simulink model "Intersection_Sim_V23"  (R2024b)
settings: Solver=VariableStepAuto  StartTime=0.0  StopTime=5  RelTol=1e-3
settings Model: Creator=nelsenyoung  LastModifiedBy=hadi

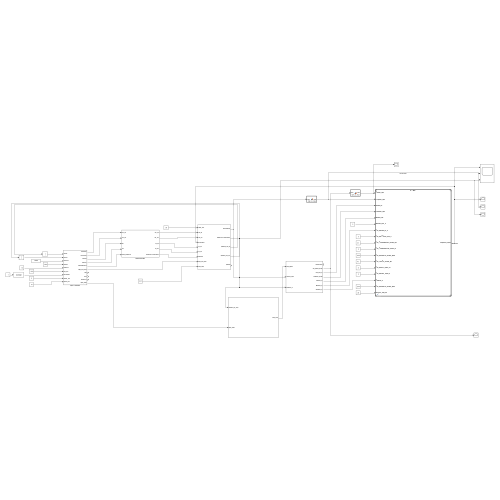
[thumbnail: Simulink's stored preview of the top-level diagram]
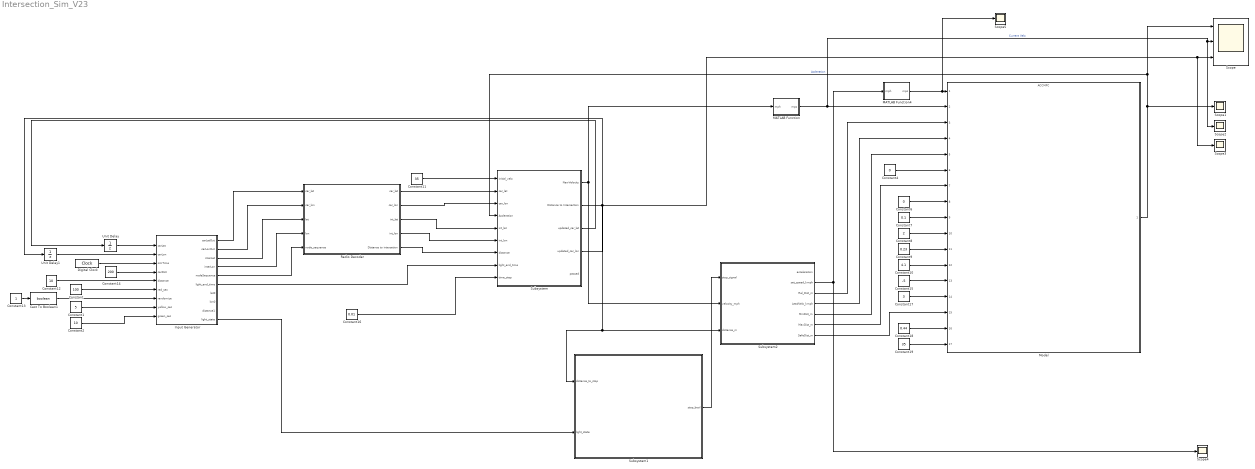
== system Intersection_Sim_V23 ==
  Cast To Boolean1 : DataTypeConversion  OutDataTypeStr=boolean  SaturateOnIntegerOverflow=off  RndMeth=Floor
  Constant : Constant  Value=100
  Constant1 : Constant  Value=5
  Constant10 : Constant  Value=4.1
  Constant11 : Constant  Value=35
  Constant12 : Constant  Value=10
  Constant13 : Constant
  Constant14 : Constant  Value=200
  Constant15 : Constant  Value=-5
  Constant16 : Constant  Value=0.01
  Constant17 : Constant  Value=3
  Constant18 : Constant  Value=0.44
  Constant19 : Constant  Value=35
  Constant2 : Constant  Value=10
  Constant4 : Constant  Value=0
  Constant6 : Constant  Value=0
  Constant7 : Constant  Value=0.1
  Constant8 : Constant  Value=2
  Constant9 : Constant  Value=0.23
  Digital Clock : DigitalClock  SampleTime=0.01
  Input Generator : Subsystem
  MATLAB Function : MATLAB Function  TreatAsAtomicUnit=on
  MATLAB Function4 : MATLAB Function  TreatAsAtomicUnit=on
  Model : ModelReference  ModelNameDialog=ACCMPC.slx  SimulationMode=Normal  ModelReferenceVersion=1.21
  Radio Decoder : Subsystem
  Scope : Scope  NumInputPorts=3
  Scope{1..5} (5 alike) : Scope
  Subsystem : Subsystem
  Subsystem1 : Subsystem
  Subsystem2 : Subsystem
  Unit Delay : UnitDelay  SampleTime=-1  HasFrameUpgradeWarning=on
  Unit Delay1 : UnitDelay  SampleTime=-1  HasFrameUpgradeWarning=on
  wires:
  Constant4/1 -> Model/6
  Constant6/1 -> Model/8
  Constant7/1 -> Model/9
  Constant8/1 -> Model/10
  Constant9/1 -> Model/11
  Constant10/1 -> Model/12
  Constant15/1 -> Model/13
  Constant17/1 -> Model/14
  Constant18/1 -> Model/16
  Constant19/1 -> Model/17
  Subsystem2/7(SafeDist_m) -> Model/15
  Model/1 -> Subsystem/4(Accleration), Scope/1, Scope1/1  "Accleration"
  MATLAB Function/1(mps) -> Scope2/1, Scope/2, Model/2  "Current Velo"
  MATLAB Function4/1(mps) -> Scope5/1, Model/1
  Constant13/1 -> Cast To Boolean1/1
  Unit Delay/1 -> Input Generator/1(carLat)
  Unit Delay1/1 -> Input Generator/2(carLon)
  Digital Clock/1 -> Input Generator/3(simTime)
  Constant14/1 -> Input Generator/4(carDist)
  Constant12/1 -> Input Generator/5(distance)
  Constant/1 -> Input Generator/6(red_sec)
  Cast To Boolean1/1 -> Input Generator/7(randomize)
  Constant1/1 -> Input Generator/8(yellow_sec)
  Constant2/1 -> Input Generator/9(green_sec)
  Input Generator/1(carLatOut) -> Radio Decoder/1("car_lat ")
  Input Generator/2(carLonOut) -> Radio Decoder/2("car_lon ")
  Input Generator/3(interLat) -> Radio Decoder/3(lat)
  Input Generator/4(interLon) -> Radio Decoder/4(lon)
  Input Generator/5(nodeSequence) -> Radio Decoder/5(node_sequence)
  Subsystem/2(Distance to Intersection) -> Scope/3, Scope3/1, Subsystem2/3(distance_m), Subsystem1/1(distance_to_stop)
  Constant11/1 -> Subsystem/1(initial_velo)
  Radio Decoder/1(car_lat) -> Subsystem/2(car_lat)
  Radio Decoder/2(car_lon) -> Subsystem/3(car_lon)
  Radio Decoder/3(int_lat) -> Subsystem/5(int_lat)
  Radio Decoder/4(int_lon) -> Subsystem/6(int_lon)
  Radio Decoder/5(Distance to intersetion) -> Subsystem/7(distance)
  Input Generator/6(light_end_time) -> Subsystem/8(light_end_time)
  Constant16/1 -> Subsystem/9(time_step)
  Subsystem/3(updated_car_lat) -> Unit Delay/1
  Subsystem/4(updated_car_lon) -> Unit Delay1/1
  Input Generator/10(light_state) -> Subsystem1/2(light_state)
  Subsystem/1(NewVelocity) -> Subsystem2/2(velocity_mph), MATLAB Function/1(mph)
  Subsystem2/2(set_speed_kmph) -> Scope4/1, MATLAB Function4/1(mph)
  Subsystem1/1(stop_bool) -> Subsystem2/1(stop_signal)
  Subsystem2/3(Rel_Dist_m) -> Model/3
  Subsystem2/4(LeadVelo_kmph) -> Model/4
  Subsystem2/5(MinDist_m) -> Model/5
  Subsystem2/6(MaxDist_m) -> Model/7

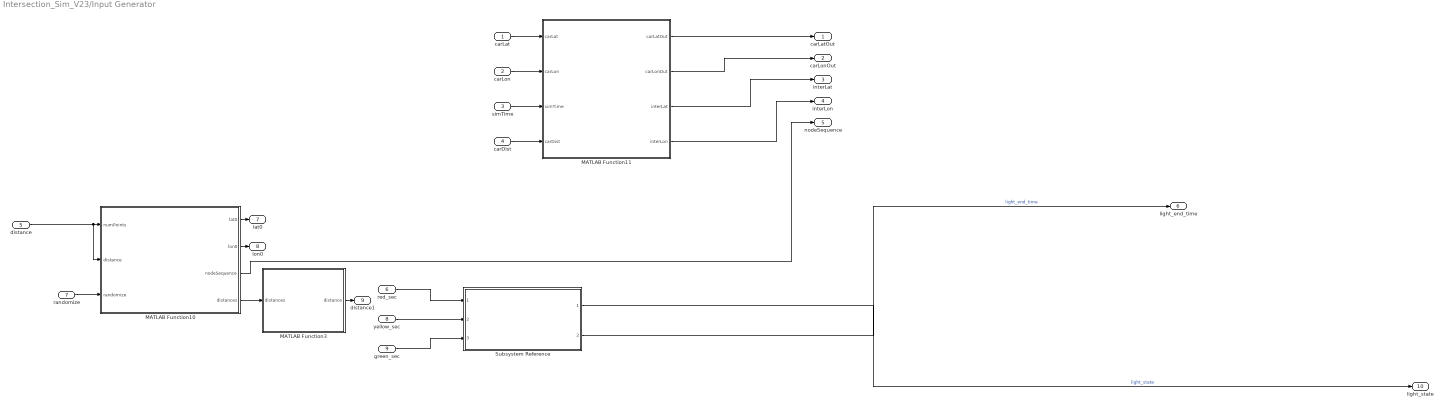
== system Intersection_Sim_V23/Input Generator ==
  carLat : Inport
  carLon : Inport  Port=2
  simTime : Inport  Port=3
  carDist : Inport  Port=4
  distance : Inport  Port=5
  red_sec : Inport  Port=6
  randomize : Inport  Port=7
  yellow_sec : Inport  Port=8
  green_sec : Inport  Port=9
  MATLAB Function10 : MATLAB Function  TreatAsAtomicUnit=on
  MATLAB Function11 : MATLAB Function  TreatAsAtomicUnit=on
  MATLAB Function3 : MATLAB Function  TreatAsAtomicUnit=on
  Subsystem Reference : Subsystem  ReferencedSubsystem=traffic_light_sim_ryg
  carLatOut : Outport
  carLonOut : Outport  Port=2
  interLat : Outport  Port=3
  interLon : Outport  Port=4
  nodeSequence : Outport  Port=5
  light_end_time : Outport  Port=6
  lat0 : Outport  Port=7
  lon0 : Outport  Port=8
  distance1 : Outport  Port=9
  light_state : Outport  Port=10
  wires:
  Subsystem Reference/1 -> light_state/1  "light_state"
  MATLAB Function11/2(carLonOut) -> carLonOut/1
  Subsystem Reference/2 -> light_end_time/1  "light_end_time"
  carLon/1 -> MATLAB Function11/2(carLon)
  MATLAB Function11/4(interLon) -> interLon/1
  MATLAB Function11/1(carLatOut) -> carLatOut/1
  MATLAB Function3/1(distance) -> distance1/1
  MATLAB Function11/3(interLat) -> interLat/1
  distance/1 -> MATLAB Function10/1(numPoints), MATLAB Function10/2(distance)
  MATLAB Function10/3(nodeSequence) -> nodeSequence/1
  MATLAB Function10/4(distances) -> MATLAB Function3/1(distances)
  MATLAB Function10/2(lon0) -> lon0/1
  red_sec/1 -> Subsystem Reference/1
  yellow_sec/1 -> Subsystem Reference/2
  simTime/1 -> MATLAB Function11/3(simTime)
  randomize/1 -> MATLAB Function10/3(randomize)
  MATLAB Function10/1(lat0) -> lat0/1
  green_sec/1 -> Subsystem Reference/3
  carLat/1 -> MATLAB Function11/1(carLat)
  carDist/1 -> MATLAB Function11/4(carDist)

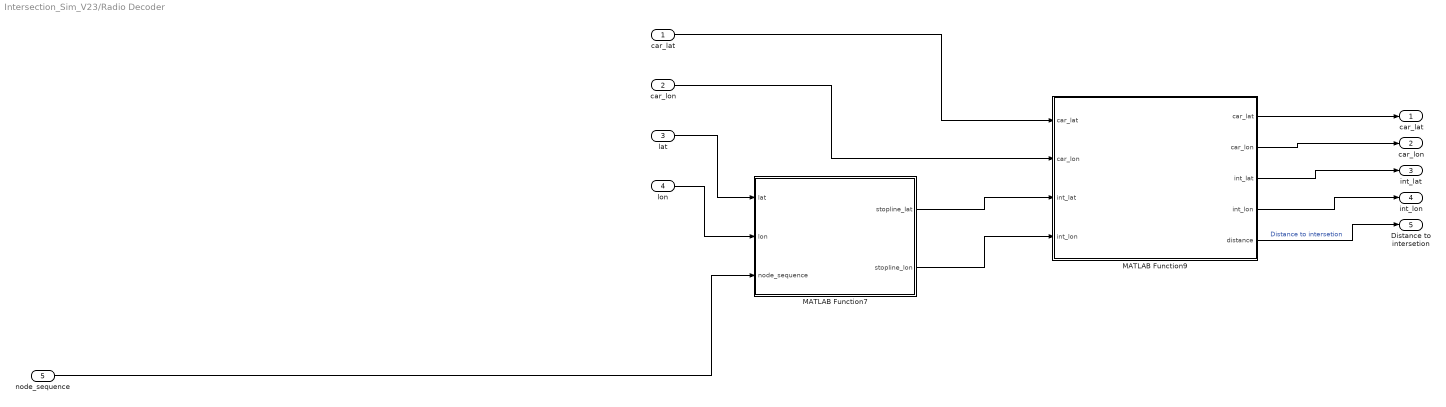
== system Intersection_Sim_V23/Radio Decoder ==
  "car_lat " : Inport
  "car_lon " : Inport  Port=2
  lat : Inport  Port=3
  lon : Inport  Port=4
  node_sequence : Inport  Port=5
  MATLAB Function7 : MATLAB Function  TreatAsAtomicUnit=on
  MATLAB Function9 : MATLAB Function  TreatAsAtomicUnit=on
  car_lat : Outport
  car_lon : Outport  Port=2
  int_lat : Outport  Port=3
  int_lon : Outport  Port=4
  Distance to intersetion : Outport  Port=5
  wires:
  "car_lat "/1 -> MATLAB Function9/1("car_lat ")
  MATLAB Function9/1(car_lat) -> car_lat/1
  MATLAB Function9/2(car_lon) -> car_lon/1
  MATLAB Function9/3(int_lat) -> int_lat/1
  MATLAB Function7/2(stopline_lon) -> MATLAB Function9/4("int_lon ")
  lat/1 -> MATLAB Function7/1(lat)
  MATLAB Function9/4(int_lon) -> int_lon/1
  lon/1 -> MATLAB Function7/2(lon)
  MATLAB Function7/1(stopline_lat) -> MATLAB Function9/3("int_lat ")
  "car_lon "/1 -> MATLAB Function9/2("car_lon ")
  node_sequence/1 -> MATLAB Function7/3(node_sequence)
  MATLAB Function9/5(distance) -> Distance to intersetion/1  "Distance to intersetion"

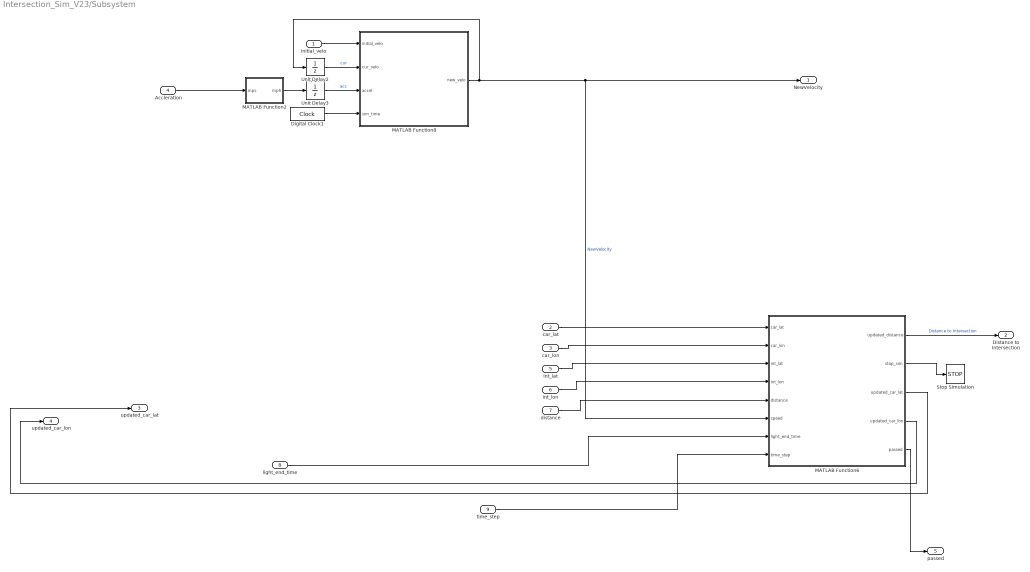
== system Intersection_Sim_V23/Subsystem ==
  initial_velo : Inport
  car_lat : Inport  Port=2
  car_lon : Inport  Port=3
  Accleration : Inport  Port=4
  int_lat : Inport  Port=5
  int_lon : Inport  Port=6
  distance : Inport  Port=7
  light_end_time : Inport  Port=8
  time_step : Inport  Port=9
  Digital Clock1 : DigitalClock  SampleTime=0.01
  MATLAB Function2 : MATLAB Function  TreatAsAtomicUnit=on
  MATLAB Function6 : MATLAB Function  TreatAsAtomicUnit=on
  MATLAB Function8 : MATLAB Function  TreatAsAtomicUnit=on
  Stop Simulation : Stop
  Unit Delay2 : UnitDelay  SampleTime=-1  HasFrameUpgradeWarning=on
  Unit Delay3 : UnitDelay  SampleTime=-1  HasFrameUpgradeWarning=on
  NewVelocity : Outport
  Distance to Intersection : Outport  Port=2
  updated_car_lat : Outport  Port=3
  updated_car_lon : Outport  Port=4
  passed : Outport  Port=5
  wires:
  int_lon/1 -> MATLAB Function6/4(int_lon)
  distance/1 -> MATLAB Function6/5(distance)
  car_lon/1 -> MATLAB Function6/2(car_lon)
  time_step/1 -> MATLAB Function6/8(time_step)
  MATLAB Function6/3(updated_car_lat) -> updated_car_lat/1
  MATLAB Function2/1(mph) -> Unit Delay3/1
  MATLAB Function6/1(updated_distance) -> Distance to Intersection/1  "Distance to Intersection"
  initial_velo/1 -> MATLAB Function8/1(initial_velo)
  Accleration/1 -> MATLAB Function2/1(mps)
  Digital Clock1/1 -> MATLAB Function8/4(sim_time)
  light_end_time/1 -> MATLAB Function6/7(light_end_time)
  car_lat/1 -> MATLAB Function6/1(car_lat)
  int_lat/1 -> MATLAB Function6/3(int_lat)
  MATLAB Function6/2(stop_sim) -> Stop Simulation/1
  Unit Delay3/1 -> MATLAB Function8/3(accel)  "acc"
  MATLAB Function8/1(new_velo) -> NewVelocity/1, MATLAB Function6/6(speed), Unit Delay2/1  "NewVelocity"
  MATLAB Function6/5(passed) -> passed/1
  MATLAB Function6/4(updated_car_lon) -> updated_car_lon/1
  Unit Delay2/1 -> MATLAB Function8/2(cur_velo)  "cur"

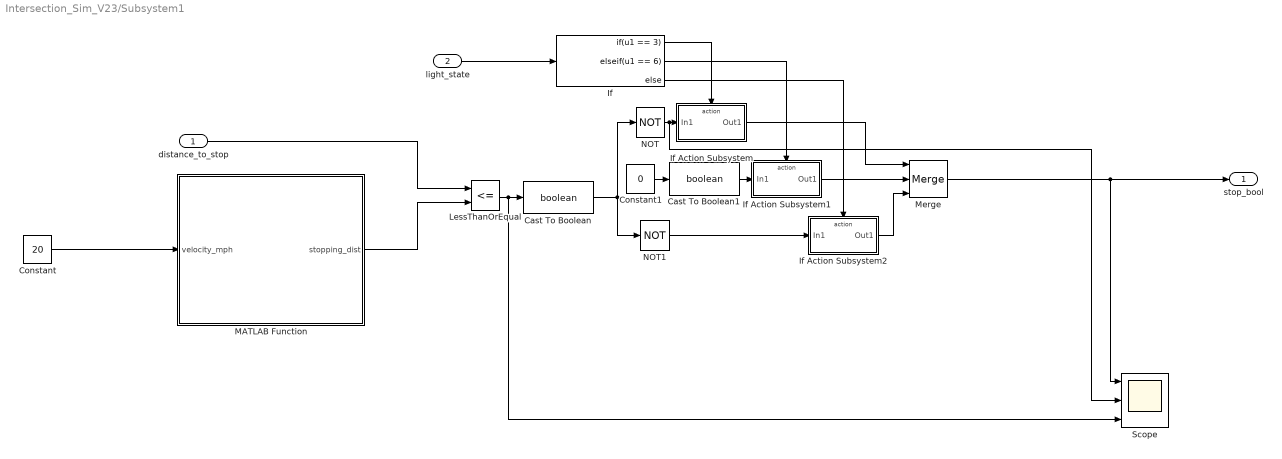
== system Intersection_Sim_V23/Subsystem1 ==
  distance_to_stop : Inport
  light_state : Inport  Port=2
  Cast To Boolean : DataTypeConversion  OutDataTypeStr=boolean  SaturateOnIntegerOverflow=off  RndMeth=Floor
  Cast To Boolean1 : DataTypeConversion  OutDataTypeStr=boolean  SaturateOnIntegerOverflow=off  RndMeth=Floor
  Constant : Constant  Value=20
  Constant1 : Constant  Value=0
  If : If  IfExpression=u1 == 3  ElseIfExpressions=u1 == 6
  If Action Subsystem : Subsystem  TreatAsAtomicUnit=on
  If Action Subsystem1 : Subsystem  TreatAsAtomicUnit=on
  If Action Subsystem2 : Subsystem  TreatAsAtomicUnit=on
  LessThanOrEqual : RelationalOperator  Operator=<=  OutDataTypeStr=boolean  RndMeth=Simplest  InputSameDT=off
  MATLAB Function : MATLAB Function  TreatAsAtomicUnit=on
  Merge : Merge  Inputs=3
  NOT : Logic  Operator=NOT  IconShape=distinctive  AllPortsSameDT=off  OutDataTypeStr=boolean
  NOT1 : Logic  Operator=NOT  IconShape=distinctive  AllPortsSameDT=off  OutDataTypeStr=boolean
  Scope : Scope  NumInputPorts=3
  stop_bool : Outport
  wires:
  Constant/1 -> MATLAB Function/1(velocity_mph)
  MATLAB Function/1(stopping_dist) -> LessThanOrEqual/2
  Merge/1 -> Scope/1, stop_bool/1
  If/1 -> If Action Subsystem/Action
  NOT/1 -> Scope/2, If Action Subsystem/1(In1)
  LessThanOrEqual/1 -> Scope/3, Cast To Boolean/1
  Cast To Boolean/1 -> NOT1/1, NOT/1
  If Action Subsystem/1(Out1) -> Merge/1
  If/2 -> If Action Subsystem1/Action
  Cast To Boolean1/1 -> If Action Subsystem1/1(In1)
  Constant1/1 -> Cast To Boolean1/1
  If Action Subsystem1/1(Out1) -> Merge/2
  If/3 -> If Action Subsystem2/Action
  NOT1/1 -> If Action Subsystem2/1(In1)
  If Action Subsystem2/1(Out1) -> Merge/3
  light_state/1 -> If/1
  distance_to_stop/1 -> LessThanOrEqual/1

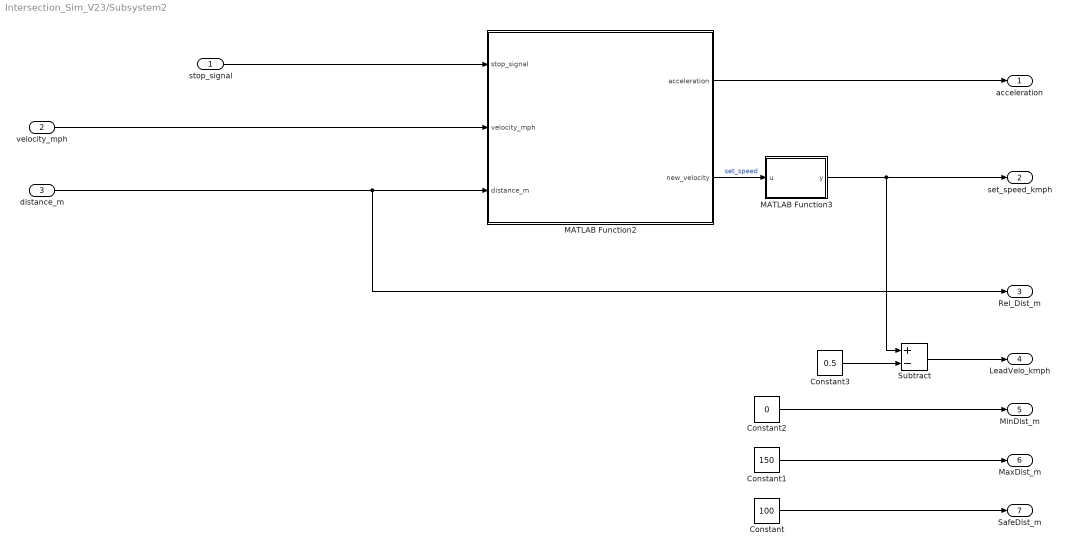
== system Intersection_Sim_V23/Subsystem2 ==
  stop_signal : Inport
  velocity_mph : Inport  Port=2
  distance_m : Inport  Port=3
  Constant : Constant  Value=100
  Constant1 : Constant  Value=150
  Constant2 : Constant  Value=0
  Constant3 : Constant  Value=0.5
  MATLAB Function2 : MATLAB Function  TreatAsAtomicUnit=on
  MATLAB Function3 : MATLAB Function  TreatAsAtomicUnit=on
  Subtract : Sum  Inputs=+-
  acceleration : Outport
  set_speed_kmph : Outport  Port=2
  Rel_Dist_m : Outport  Port=3
  LeadVelo_kmph : Outport  Port=4
  MinDist_m : Outport  Port=5
  MaxDist_m : Outport  Port=6
  SafeDist_m : Outport  Port=7
  wires:
  distance_m/1 -> Rel_Dist_m/1, MATLAB Function2/3(distance_m)
  stop_signal/1 -> MATLAB Function2/1(stop_signal)
  MATLAB Function2/1(acceleration) -> acceleration/1
  velocity_mph/1 -> MATLAB Function2/2(velocity_mph)
  MATLAB Function2/2(new_velocity) -> MATLAB Function3/1(u)  "set_speed"
  MATLAB Function3/1(y) -> Subtract/1, set_speed_kmph/1
  Constant/1 -> SafeDist_m/1
  Constant1/1 -> MaxDist_m/1
  Constant2/1 -> MinDist_m/1
  Subtract/1 -> LeadVelo_kmph/1
  Constant3/1 -> Subtract/2

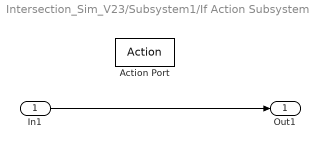
== system Intersection_Sim_V23/Subsystem1/If Action Subsystem ==
  In1 : Inport
  Action Port : ActionPort  ActionPortLabel=if(u1 == 3)
  Out1 : Outport
  wires:
  In1/1 -> Out1/1

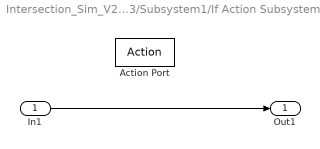
== system Intersection_Sim_V23/Subsystem1/If Action Subsystem1 ==
  In1 : Inport
  Action Port : ActionPort  ActionPortLabel=elseif(u1 == 6)
  Out1 : Outport
  wires:
  In1/1 -> Out1/1

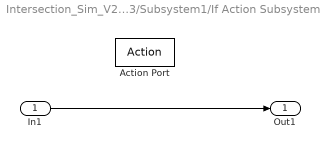
== system Intersection_Sim_V23/Subsystem1/If Action Subsystem2 ==
  In1 : Inport
  Action Port : ActionPort  ActionPortLabel=else
  Out1 : Outport
  wires:
  In1/1 -> Out1/1

== matlab function Intersection_Sim_V23/Input Generator/MATLAB Function10 ==
  data: lat0 output; lon0 output; numPoints input; distance input; randomize input; nodeSequence output; distances output
function [lat0, lon0, nodeSequence, distances] = generateNodeXY(numPoints, distance, randomize)
    % GENERATENODEXY Generates a sequence of node points for a path.
    % This function initializes once at the start of the Simulink simulation
    % and retains the same values throughout the simulation.
    %
    % INPUTS:
    %   numPoints  - Number of points in the path (integer, max 63)
    %   distance   - Distance between points (meters, scalar)
    %   randomize  - Boolean flag to randomize distance between 2-50m
    %
    % OUTPUTS:
    %   lat0        - Initial latitude
    %   lon0        - Initial longitude
    %   nodeSequence - numPoints x 2 matrix with node distances and angles
    %   distances   - Array of Euclidean distances between nodes

    % Define persistent variables
    persistent initialized lat0_p lon0_p nodeSequence_p distances_p
    
    numPoints = 3;

    % If not initialized, generate values
    if isempty(initialized)
        initialized = true;  % Set flag to indicate initialization

        % Validate inputs
        if numPoints < 2 || numPoints > 63
            error('Number of points must be between 2 and 63.');
        end

        % Generate a random starting point (latitude and longitude)
        lat0_p = -90 + (180 * rand); % Random latitude (-90 to 90)
        lon0_p = -180 + (360 * rand); % Random longitude (-180 to 180)

        % Initialize node sequence
        nodeSequence_p = zeros(numPoints, 2);
        nodeSequence_p(1, :) = [lat0_p, lon0_p];

        % Initialize distances
        distances_p = zeros(numPoints, 1);
        distances_p(1) = 0;

        for i = 2:numPoints
            if randomize
                x = 2 + (50 - 2) * rand; % Random distance between 2m and 50m
            else
                x = distance;
            end

            if randomize
                y = 2 + (50 - 2) * rand;
            else
                y = distance;
            end

            % Store distances
            nodeSequence_p(i, 1) = x;
            nodeSequence_p(i, 2) = y;
            distances_p(i) = sqrt((x*x) + (y*y));
        end
    end

    % Output the persistent values
    lat0 = lat0_p;
    lon0 = lon0_p;
    nodeSequence = nodeSequence_p;
    distances = distances_p;
end

== matlab function Intersection_Sim_V23/Input Generator/MATLAB Function11 ==
  data: carLat input; carLatOut output; carLon input; simTime input; carDist input; carLonOut output; interLat output; interLon output
function [carLatOut, carLonOut, interLat, interLon] = car_position_update(carLat, carLon, simTime, carDist)
    % Define Earth's radius in meters
    R = 6371000;
    
    % Persistent variables to store intersection coordinates
    persistent interLatStored interLonStored;
    
    % Generate random intersection coordinates only once at simulation start
    if isempty(interLatStored) || isempty(interLonStored)
        interLatStored = -90 + (rand * 180); % Random latitude between -90 and 90 degrees
        interLonStored = -180 + (rand * 360); % Random longitude between -180 and 180 degrees
    end
    
    interLat = interLatStored;
    interLon = interLonStored;
    
    % Generate a car position at a given distance from the intersection at a random bearing
    bearing = rand * 2 * pi; % Random bearing in radians
    
    % Convert distance from meters to degrees
    deltaLatDist = (carDist / R) * (180 / pi);
    deltaLonDist = (carDist / R) * (180 / pi) / cos(interLat * pi / 180);
    
    % Calculate new latitude
    newLat = interLat + deltaLatDist * cos(bearing);
    
    % Calculate new longitude
    newLon = interLon + deltaLonDist * sin(bearing);
    
    % If simulation time is less than 0.1, use the generated car position
    if simTime < 0.01
        carLatOut = newLat;
        carLonOut = newLon;
    else
        carLatOut = carLat;
        carLonOut = carLon;
    end
end

== matlab function Intersection_Sim_V23/Subsystem1/MATLAB Function ==
  data: velocity_mph input; stopping_dist output
function stopping_dist = stopping_distance(velocity_mph)
    % Stopping Distance Calculation for Simulink
    % 
    % velocity_mph: Velocity in miles per hour (0 to 35 mph)
    % stopping_dist: Stopping distance in meters
    %
    % Ensure velocity is within the valid range
    if velocity_mph < 0 || velocity_mph > 35
        error('Velocity must be between 0 and 35 mph.');
    end
    
    % Constants
    deceleration = 2.8; % m/s^2
    mph_to_mps = 0.44704; % Conversion factor from mph to m/s
    
    % Convert velocity from mph to m/s
    velocity_mps = velocity_mph * mph_to_mps;
    
    % Use kinematic equation: d = v^2 / (2 * a)
    stopping_dist = (velocity_mps ^ 2) / (2 * deceleration);
end

== matlab function Intersection_Sim_V23/Subsystem2/MATLAB Function2 ==
  data: acceleration output; stop_signal input; new_velocity output; velocity_mph input; distance_m input
function [acceleration, new_velocity] = calculate_acceleration(stop_signal, velocity_mph, distance_m)
    % Calculate required acceleration to stop at a given distance
    %
    % stop_signal: Boolean (0 = go, 1 = stop)
    % velocity_mph: Current velocity in miles per hour (0 to 35 mph)
    % distance_m: Distance available to stop in meters
    % acceleration: Required acceleration in m/s^2 (negative for deceleration)
    % new_velocity: Adjusted velocity after applying calculated acceleration
    
    % Constants
    mph_to_mps = 0.44704; % Conversion factor from mph to m/s
    
    % Convert velocity from mph to m/s
    velocity_mps = velocity_mph * mph_to_mps;
    
    if stop_signal == 1
        % Use kinematic equation: v^2 = u^2 + 2as => a = -u^2 / (2 * s)
        if distance_m > 0
            acceleration = - (velocity_mps ^ 2) / (2 * distance_m);
        else
            acceleration = -inf; % Instant stop required, not feasible
        end
        
        % Compute the new velocity after applying acceleration
        new_velocity = velocity_mps + acceleration;
    else
        % If stop_signal is 0 (go), maintain current velocity with zero acceleration
        acceleration = 0;
        new_velocity = velocity_mps;
    end
    
    % Convert new velocity back to mph
    new_velocity = new_velocity / mph_to_mps;
end

== matlab function Intersection_Sim_V23/Subsystem/MATLAB Function6 ==
  data: car_lat input; car_lon input; int_lat input; int_lon input; distance input; updated_distance output; stop_sim output; speed input; light_end_time input; time_step input; updated_car_lat output; updated_car_lon output; passed output
function [updated_distance, stop_sim, updated_car_lat, updated_car_lon, passed] = update_distance_to_intersection(car_lat, car_lon, int_lat, int_lon, distance, speed, light_end_time, time_step)
    % Convert speed from miles per hour to meters per second
    speed_in_meters = speed / 2.237; 
    
    % Calculate the change in distance traveled by the car
    distance_traveled = speed_in_meters * time_step;
    
    % Calculate the direction of movement towards the intersection
    % First, calculate the unit vector pointing from the car to the intersection
    delta_lat = int_lat - car_lat;
    delta_lon = int_lon - car_lon;
    angle = atan2(delta_lat, delta_lon);
    
    % Update the car's position
    updated_car_lat = car_lat + (distance_traveled / distance) * delta_lat;
    updated_car_lon = car_lon + (distance_traveled / distance) * delta_lon;
    
    % Calculate the updated distance to the intersection
    updated_distance = distance - distance_traveled;
    
    stop_sim = false;
    if updated_distance <= 0
        stop_sim = true;
    end

    % Check if we pass the intersection by the time the light ends
    distance_traveld_before_light_end = speed_in_meters * light_end_time;
    passed = false;
    if (distance - distance_traveld_before_light_end) <= 0
        passed = true;
    end
end

== matlab function Intersection_Sim_V23/MATLAB Function ==
  data: mph input; mps output
function mps = mph_to_mps(mph)
%MPH_TO_MPS Converts speed from miles per hour to meters per second
%   Input:
%       mph - Speed in miles per hour
%   Output:
%       mps - Speed in meters per second

    % Conversion factor (1 mph = 0.44704 mps)
    conversion_factor = 0.44704;
    
    % Convert mph to mps
    mps = mph * conversion_factor;
end

== matlab function Intersection_Sim_V23/Subsystem2/MATLAB Function3 ==
  data: u input; y output
function y = fcn(u)
    if u == 0
        y = 35;
    else
        y = 0;
    end
end

== matlab function Intersection_Sim_V23/Radio Decoder/MATLAB Function7 ==
  data: lat input; lon input; node_sequence input; stopline_lat output; stopline_lon output
function [stopline_lat, stopline_lon] = calculate_stopline_from_sequence(lat, lon, node_sequence)
    x_offset = 0;
    y_offset = 0;

    for i = 2:3
        x = node_sequence(i, 1);
        y = node_sequence(i, 2);

        % Sum the distances in both directions
        x_offset = x_offset + x;
        y_offset = y_offset + y;
    end

    % Earth's radius in meters
    R = 6378137;  

    % Convert latitude and longitude from degrees to radians
    lat_rad = deg2rad(lat);
    lon_rad = deg2rad(lon);

    % Calculate new latitude (y direction)
    new_lat_rad = lat_rad + (y_offset / R);

    % Calculate new longitude (x direction), accounting for latitude
    new_lon_rad = lon_rad + (x_offset / (R * cos(lat_rad)));

    % Convert back to degrees
    stopline_lat = rad2deg(new_lat_rad);
    stopline_lon = rad2deg(new_lon_rad);
end

== matlab function Intersection_Sim_V23/Input Generator/MATLAB Function3 ==
  data: distances input; distance output
function distance = fold_sum_vector(distances)

    distance = sum(distances);
end

== matlab function Intersection_Sim_V23/Subsystem/MATLAB Function2 ==
  data: mps input; mph output
function mph = mps_to_mph(mps)
%MPS_TO_MPH Converts speed from meters per second to miles per hour
%   Input:
%       mps - Speed in meters per second
%   Output:
%       mph - Speed in miles per hour

    % Conversion factor (1 mps = 2.23694 mph)
    conversion_factor = 2.23694;
    
    % Convert mps to mph
    mph = mps * conversion_factor;
end

== matlab function Intersection_Sim_V23/MATLAB Function4 ==
  data: mph input; mps output
function mps = mph_to_mps(mph)
%MPH_TO_MPS Converts speed from miles per hour to meters per second
%   Input:
%       mph - Speed in miles per hour
%   Output:
%       mps - Speed in meters per second

    % Conversion factor (1 mph = 0.44704 mps)
    conversion_factor = 0.44704;
    
    % Convert mph to mps
    mps = mph * conversion_factor;
end

== matlab function Intersection_Sim_V23/Subsystem/MATLAB Function8 ==
  data: initial_velo input; cur_velo input; new_velo output; accel input; sim_time input
function new_velo = update_velocity(initial_velo, cur_velo, accel, sim_time)
    if sim_time < 0.01
        cur_velo = initial_velo;
    end
    new_velo = cur_velo + accel;
end

== matlab function Intersection_Sim_V23/Radio Decoder/MATLAB Function9 ==
  data: car_lat output; car_lon output; int_lat output; int_lon output; car_lat input; distance output; car_lon input; int_lat input; int_lon input
function [car_lat, car_lon, int_lat, int_lon, distance] = haversine_distance(car_lat, car_lon, int_lat, int_lon)
    % haversine_distance calculates the distance between two points
    % on the Earth's surface given their latitude and longitude in degrees.
    % The result is in meters.

    % Radius of the Earth in meters
    R = 6371000; 
    
    % Convert latitude and longitude from degrees to radians
    car_lat = deg2rad(car_lat);
    car_lon = deg2rad(car_lon);
    int_lat = deg2rad(int_lat);
    int_lon = deg2rad(int_lon);
    
    % Haversine formula
    dlat = int_lat - car_lat;
    dlon = int_lon - car_lon;
    
    a = sin(dlat/2)^2 + cos(car_lat) * cos(int_lat) * sin(dlon/2)^2;
    c = 2 * atan2(sqrt(a), sqrt(1-a));
    
    % Distance in meters
    distance = R * c;

    % Change coords back to degrees
    car_lat = rad2deg(car_lat);
    car_lon = rad2deg(car_lon);
    int_lat = rad2deg(int_lat);
    int_lon = rad2deg(int_lon);
end
